simulink model "Model01_3"  (R2018a)
settings: Solver=VariableStepAuto  StartTime=0.0  StopTime=10.0  RelTol=1e-3
undefined symbols (not defined in the file or in its folder): C13, I10, r, R11, R14
settings Model: Creator=ameli  LastModifiedBy=ameli

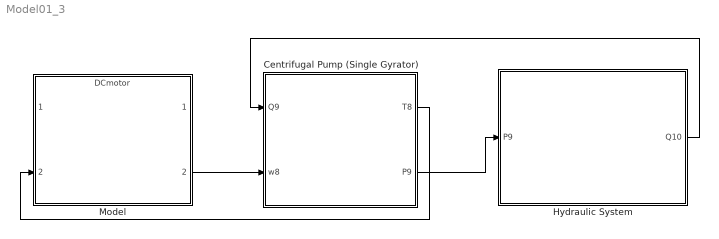
== system Model01_3 ==
  Centrifugal Pump (Single Gyrator) : Subsystem
  Hydraulic System : Subsystem
  Model : ModelReference  ModelNameDialog=DCmotor.slx  ModelReferenceVersion=1.12
  wires:
  Model/2 -> Centrifugal Pump (Single Gyrator)/2(w8)
  Centrifugal Pump (Single Gyrator)/1(T8) -> Model/2
  Centrifugal Pump (Single Gyrator)/2(P9) -> Hydraulic System/1(P9)
  Hydraulic System/1(Q10) -> Centrifugal Pump (Single Gyrator)/1(Q9)

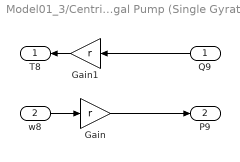
== system Model01_3/Centrifugal Pump (Single Gyrator) ==
  Q9 : Inport
  w8 : Inport  Port=2
  Gain : Gain  Gain=r
  Gain1 : Gain  Gain=r
  T8 : Outport
  P9 : Outport  Port=2
  wires:
  Gain1/1 -> T8/1
  Q9/1 -> Gain1/1
  w8/1 -> Gain/1
  Gain/1 -> P9/1

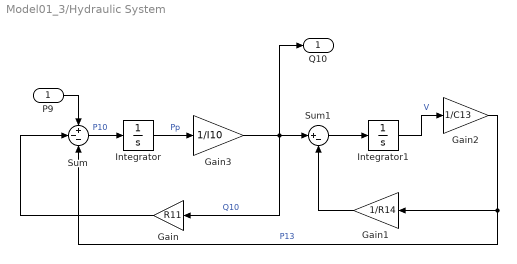
== system Model01_3/Hydraulic System ==
  P9 : Inport
  Gain : Gain  Gain=R11
  Gain1 : Gain  Gain=1/R14
  Gain2 : Gain  Gain=1/C13
  Gain3 : Gain  Gain=1/I10
  Integrator : Integrator
  Integrator1 : Integrator
  Sum : Sum  Inputs=+--
  Sum1 : Sum  Inputs=|+-
  Q10 : Outport
  wires:
  P9/1 -> Sum/1
  Sum/1 -> Integrator/1  "P10"
  Gain/1 -> Sum/2
  Integrator/1 -> Gain3/1  "Pp"
  Gain3/1 -> Gain/1, Q10/1, Sum1/1  "Q10"
  Gain1/1 -> Sum1/2
  Sum1/1 -> Integrator1/1
  Gain2/1 -> Sum/3, Gain1/1  "P13"
  Integrator1/1 -> Gain2/1  "V"
